simulink model "IEEE34_SPSload"  (R2021b)
settings: Solver=ode4  StartTime=0.0  StopTime=5  FixedStep=50e-6  RelTol=1e-3
PreLoadFcn:
  | pGain = 0.05; % Gain of random perturbation (pu)
  | pGainAP = 0.01; % Gain of sinusoidal active power variation (pu)
  | pGainRP = 0.01; % Gain of sinusoidal reactive power variation (pu)
  | pFreqAP = 0.03; % Frequency of sinusoidal active power variation (Hz)
  | pFreqRP = 0.03; % Frequency of sinusoidal reactive power variation (Hz)
  | 
  | init_IEEE34nodetestfeeder;
InitFcn:
  | pGain = 0.05; % Gain of random perturbation (pu)
  | pGainAP = 0.01; % Gain of sinusoidal active power variation (pu)
  | pGainRP = 0.01; % Gain of sinusoidal reactive power variation (pu)
  | pFreqAP = 0.03; % Frequency of sinusoidal active power variation (Hz)
  | pFreqRP = 0.03; % Frequency of sinusoidal reactive power variation (Hz)
  | 
  | init_IEEE34nodetestfeeder;
values from neighbouring files (symbols this model uses):
  fNom = f    (= 60)    [init_IEEE34nodetestfeeder.m]
  loadcoeff = 1.0    (= 1)    [init_IEEE34nodetestfeeder.m]
  Ts = 50e-6    (= 5e-05)    [init_IEEE34nodetestfeeder.m]
  vNomMV = VsubL    (= 24900)    [init_IEEE34nodetestfeeder.m]
  VsubL = 24.9e3    (= 24900)    [init_IEEE34nodetestfeeder.m]
  VxfmL = 4.16e3    (= 4160)    [init_IEEE34nodetestfeeder.m]
undefined symbols (not defined in the file or in its folder): Ac, Bc, Cc, Dc, find_system, j
libraries: spsSeriesRLCBranchLib x418, spsGroundLib x242, simulink_extras x176, spsVoltageMeasurementLib x106, spsRMSLib x96, spsControlledCurrentSourceLib x94, spsThreePhaseVIMeasurementLib x37, spsMutualInductanceLib x24, spsCurrentMeasurementLib x12, spsOnDelayLib x12, spsLinearTransformerLib x6, spsControlledVoltageSourceLib x6
(part 5 of 33)

== system IEEE34_SPSload/SM_IEEE34/DL836-1 ==
  Load B : Subsystem  DialogController=POWERSYS.PowerSysDialog  mask(Single-Phase Dynamic Load){NominalVoltage=[ VsubL 60 ], ActiveReactivePowers=[18*1000*loadcoeff 9*1000*loadcoeff]/2, PositiveSequence=[1 0], ExternalControl=off, NpNq=[1 1], TimeConstants=[0  0  0  0], MinimumVoltage=0.7, LoadFlowParameters=[4,0,0,0,0]}
      mask prompts: NominalVoltage "Nominal voltage and frequency  [Vn(Vrms) fn(Hz)]:"; ActiveReactivePowers "Active and reactive power at initial voltage [Po(W) Qo(var)]:"; PositiveSequence "Initial voltage Vo [Mag(pu) Phase (deg.)]:"; ExternalControl "External control of PQ"; NpNq "Parameters [ np  nq ]:"; TimeConstants "Time constants [Tp1 Tp2 Tq1 Tq2]  (s):"; MinimumVoltage "Minimum voltage Vmin (pu):"; LoadFlowParameters "Load Flow parameters"
      mask help:
      | Implements a single-phase dynamic load. Active  power P and reactive
      | power Q absorbed by the load vary as function of voltage V  according to the
      | following equations:
      |
      |   If V>Vmin, P and Q vary as follows:
      |        P = Po * (V/Vo)^np * (1+Tp1.s)/(1+Tp2.s)
      |        Q = Qo * (V/Vo)^nq * (1+Tq1.s)/(1+Tq2.s)
      |   if V<Vmin
      |      Same equations with np=nq=2 (constant impedance load)
      mask init:
      | block = gcb;
      | Ts = 50e-6;
      | %
      | Vnom=NominalVoltage(1); 
      | fnom=NominalVoltage(2);
      | P0=ActiveReactivePowers(1);
      | Q0=ActiveReactivePowers(2);
      | Mag_V0=PositiveSequence(1); 
      | Pha_V0=PositiveSequence(2);
      | V0_d=Mag_V0*cos(Pha_V0*pi/180);
      | V0_q=Mag_V0*sin(Pha_V0*pi/180);
      | np=NpNq(1);
      | nq=NpNq(2);
      | Tp1=TimeConstants(1); 
      | Tp2=TimeConstants(2); 
      | Tq1=TimeConstants(3); 
      | Tq2=TimeConstants(4);
      | Vbase=Vnom/sqrt(3)*sqrt(2);
      | % initial value of positive-sequence current I1
      | I1_init=(P0-j*Q0)/((V0_d-j*V0_q)*Vnom)/sqrt(3)*sqrt(2);
      | Mag_ia=abs(I1_init);
      | Phase_ia=angle(I1_init)*180/pi;
      | %
      | Vmin=MinimumVoltage;
      | PQext=ExternalControl;
      | a=exp(j*2*pi/3);
      | power_initmask();
      mask Help: helpview(psbhelp)
      mask Callback ExternalControl: powericon('ThreePhaseDynamicLoadCback',gcb);
      mask Display:
      | plot(-45,-45,45,45,[0,9,18,24,29,30,29,24,18,9,0,-9,-18,-24,-29,-30,-29,-24,-18,-9,0]*.9,[30,29,24,18,9,0,-9,-18,-24,-29,-30,-29,-24,-18,-9,0,9,18,24,29,30]*.9)
      | plot([0,0,10,0,-10,0]*1.1,[15,-5,-5,-15,-5,-5]*1.1)
  Load B1 : Subsystem  DialogController=POWERSYS.PowerSysDialog  mask(Single-Phase Dynamic Load){NominalVoltage=[ VsubL 60 ], ActiveReactivePowers=[22*1000*loadcoeff 11*1000*loadcoeff]/2, PositiveSequence=[1 0], ExternalControl=off, NpNq=[1 1], TimeConstants=[0  0  0  0], MinimumVoltage=0.7, LoadFlowParameters=[4,0,0,0,0]}
      mask prompts: NominalVoltage "Nominal voltage and frequency  [Vn(Vrms) fn(Hz)]:"; ActiveReactivePowers "Active and reactive power at initial voltage [Po(W) Qo(var)]:"; PositiveSequence "Initial voltage Vo [Mag(pu) Phase (deg.)]:"; ExternalControl "External control of PQ"; NpNq "Parameters [ np  nq ]:"; TimeConstants "Time constants [Tp1 Tp2 Tq1 Tq2]  (s):"; MinimumVoltage "Minimum voltage Vmin (pu):"; LoadFlowParameters "Load Flow parameters"
      mask help:
      | Implements a single-phase dynamic load. Active  power P and reactive
      | power Q absorbed by the load vary as function of voltage V  according to the
      | following equations:
      |
      |   If V>Vmin, P and Q vary as follows:
      |        P = Po * (V/Vo)^np * (1+Tp1.s)/(1+Tp2.s)
      |        Q = Qo * (V/Vo)^nq * (1+Tq1.s)/(1+Tq2.s)
      |   if V<Vmin
      |      Same equations with np=nq=2 (constant impedance load)
      mask init: same as IEEE34_SPSload/SM_IEEE34/DL836-1/Load B
      mask Help: helpview(psbhelp)
      mask Callback ExternalControl: powericon('ThreePhaseDynamicLoadCback',gcb);
      mask Display:
      | plot(-45,-45,45,45,[0,9,18,24,29,30,29,24,18,9,0,-9,-18,-24,-29,-30,-29,-24,-18,-9,0]*.9,[30,29,24,18,9,0,-9,-18,-24,-29,-30,-29,-24,-18,-9,0,9,18,24,29,30]*.9)
      | plot([0,0,10,0,-10,0]*1.1,[15,-5,-5,-15,-5,-5]*1.1)
  Load B2 : Subsystem  DialogController=POWERSYS.PowerSysDialog  mask(Single-Phase Dynamic Load){NominalVoltage=[ VsubL 60 ], ActiveReactivePowers=[1e-6*1000*loadcoeff 0*1000*loadcoeff]/2, PositiveSequence=[1 0], ExternalControl=off, NpNq=[1 1], TimeConstants=[0  0  0  0], MinimumVoltage=0.7, LoadFlowParameters=[4,0,0,0,0]}
      mask prompts: NominalVoltage "Nominal voltage and frequency  [Vn(Vrms) fn(Hz)]:"; ActiveReactivePowers "Active and reactive power at initial voltage [Po(W) Qo(var)]:"; PositiveSequence "Initial voltage Vo [Mag(pu) Phase (deg.)]:"; ExternalControl "External control of PQ"; NpNq "Parameters [ np  nq ]:"; TimeConstants "Time constants [Tp1 Tp2 Tq1 Tq2]  (s):"; MinimumVoltage "Minimum voltage Vmin (pu):"; LoadFlowParameters "Load Flow parameters"
      mask help:
      | Implements a single-phase dynamic load. Active  power P and reactive
      | power Q absorbed by the load vary as function of voltage V  according to the
      | following equations:
      |
      |   If V>Vmin, P and Q vary as follows:
      |        P = Po * (V/Vo)^np * (1+Tp1.s)/(1+Tp2.s)
      |        Q = Qo * (V/Vo)^nq * (1+Tq1.s)/(1+Tq2.s)
      |   if V<Vmin
      |      Same equations with np=nq=2 (constant impedance load)
      mask init: same as IEEE34_SPSload/SM_IEEE34/DL836-1/Load B
      mask Help: helpview(psbhelp)
      mask Callback ExternalControl: powericon('ThreePhaseDynamicLoadCback',gcb);
      mask Display:
      | plot(-45,-45,45,45,[0,9,18,24,29,30,29,24,18,9,0,-9,-18,-24,-29,-30,-29,-24,-18,-9,0]*.9,[30,29,24,18,9,0,-9,-18,-24,-29,-30,-29,-24,-18,-9,0,9,18,24,29,30]*.9)
      | plot([0,0,10,0,-10,0]*1.1,[15,-5,-5,-15,-5,-5]*1.1)
  Terminator : Terminator
  Terminator1 : Terminator
  A : PMIOPort  Side=Right
  B : PMIOPort  Port=2  Side=Right
  C : PMIOPort  Port=3  Side=Right
  wires:
  Load B1/1(m) -> Terminator1/1
  Load B/1(m) -> Terminator/1
  connections:
  C/RConn1 -- Load B1/LConn2 -- Load B2/LConn1
  Load B1/LConn1 -- Load B/LConn2 -- B/RConn1
  Load B/LConn1 -- Load B2/LConn2 -- A/RConn1

== system IEEE34_SPSload/SM_IEEE34/DL836-840 ==
  Load B : Subsystem  DialogController=POWERSYS.PowerSysDialog  mask(Single-Phase Dynamic Load){NominalVoltage=[ VsubL 60 ], ActiveReactivePowers=[18*1000*loadcoeff 9*1000*loadcoeff]/2, PositiveSequence=[1 0], ExternalControl=off, NpNq=[1 1], TimeConstants=[0  0  0  0], MinimumVoltage=0.7, LoadFlowParameters=[4,0,0,0,0]}
      mask prompts: NominalVoltage "Nominal voltage and frequency  [Vn(Vrms) fn(Hz)]:"; ActiveReactivePowers "Active and reactive power at initial voltage [Po(W) Qo(var)]:"; PositiveSequence "Initial voltage Vo [Mag(pu) Phase (deg.)]:"; ExternalControl "External control of PQ"; NpNq "Parameters [ np  nq ]:"; TimeConstants "Time constants [Tp1 Tp2 Tq1 Tq2]  (s):"; MinimumVoltage "Minimum voltage Vmin (pu):"; LoadFlowParameters "Load Flow parameters"
      mask help:
      | Implements a single-phase dynamic load. Active  power P and reactive
      | power Q absorbed by the load vary as function of voltage V  according to the
      | following equations:
      |
      |   If V>Vmin, P and Q vary as follows:
      |        P = Po * (V/Vo)^np * (1+Tp1.s)/(1+Tp2.s)
      |        Q = Qo * (V/Vo)^nq * (1+Tq1.s)/(1+Tq2.s)
      |   if V<Vmin
      |      Same equations with np=nq=2 (constant impedance load)
      mask init: same as IEEE34_SPSload/SM_IEEE34/DL836-1/Load B
      mask Help: helpview(psbhelp)
      mask Callback ExternalControl: powericon('ThreePhaseDynamicLoadCback',gcb);
      mask Display:
      | plot(-45,-45,45,45,[0,9,18,24,29,30,29,24,18,9,0,-9,-18,-24,-29,-30,-29,-24,-18,-9,0]*.9,[30,29,24,18,9,0,-9,-18,-24,-29,-30,-29,-24,-18,-9,0,9,18,24,29,30]*.9)
      | plot([0,0,10,0,-10,0]*1.1,[15,-5,-5,-15,-5,-5]*1.1)
  Load B1 : Subsystem  DialogController=POWERSYS.PowerSysDialog  mask(Single-Phase Dynamic Load){NominalVoltage=[ VsubL 60 ], ActiveReactivePowers=[22*1000*loadcoeff 11*1000*loadcoeff]/2, PositiveSequence=[1 0], ExternalControl=off, NpNq=[1 1], TimeConstants=[0  0  0  0], MinimumVoltage=0.7, LoadFlowParameters=[4,0,0,0,0]}
      mask prompts: NominalVoltage "Nominal voltage and frequency  [Vn(Vrms) fn(Hz)]:"; ActiveReactivePowers "Active and reactive power at initial voltage [Po(W) Qo(var)]:"; PositiveSequence "Initial voltage Vo [Mag(pu) Phase (deg.)]:"; ExternalControl "External control of PQ"; NpNq "Parameters [ np  nq ]:"; TimeConstants "Time constants [Tp1 Tp2 Tq1 Tq2]  (s):"; MinimumVoltage "Minimum voltage Vmin (pu):"; LoadFlowParameters "Load Flow parameters"
      mask help:
      | Implements a single-phase dynamic load. Active  power P and reactive
      | power Q absorbed by the load vary as function of voltage V  according to the
      | following equations:
      |
      |   If V>Vmin, P and Q vary as follows:
      |        P = Po * (V/Vo)^np * (1+Tp1.s)/(1+Tp2.s)
      |        Q = Qo * (V/Vo)^nq * (1+Tq1.s)/(1+Tq2.s)
      |   if V<Vmin
      |      Same equations with np=nq=2 (constant impedance load)
      mask init: same as IEEE34_SPSload/SM_IEEE34/DL836-1/Load B
      mask Help: helpview(psbhelp)
      mask Callback ExternalControl: powericon('ThreePhaseDynamicLoadCback',gcb);
      mask Display:
      | plot(-45,-45,45,45,[0,9,18,24,29,30,29,24,18,9,0,-9,-18,-24,-29,-30,-29,-24,-18,-9,0]*.9,[30,29,24,18,9,0,-9,-18,-24,-29,-30,-29,-24,-18,-9,0,9,18,24,29,30]*.9)
      | plot([0,0,10,0,-10,0]*1.1,[15,-5,-5,-15,-5,-5]*1.1)
  Load B2 : Subsystem  DialogController=POWERSYS.PowerSysDialog  mask(Single-Phase Dynamic Load){NominalVoltage=[ VsubL 60 ], ActiveReactivePowers=[1e-6*1000*loadcoeff 0*1000*loadcoeff]/2, PositiveSequence=[1 0], ExternalControl=off, NpNq=[1 1], TimeConstants=[0  0  0  0], MinimumVoltage=0.7, LoadFlowParameters=[4,0,0,0,0]}
      mask prompts: NominalVoltage "Nominal voltage and frequency  [Vn(Vrms) fn(Hz)]:"; ActiveReactivePowers "Active and reactive power at initial voltage [Po(W) Qo(var)]:"; PositiveSequence "Initial voltage Vo [Mag(pu) Phase (deg.)]:"; ExternalControl "External control of PQ"; NpNq "Parameters [ np  nq ]:"; TimeConstants "Time constants [Tp1 Tp2 Tq1 Tq2]  (s):"; MinimumVoltage "Minimum voltage Vmin (pu):"; LoadFlowParameters "Load Flow parameters"
      mask help:
      | Implements a single-phase dynamic load. Active  power P and reactive
      | power Q absorbed by the load vary as function of voltage V  according to the
      | following equations:
      |
      |   If V>Vmin, P and Q vary as follows:
      |        P = Po * (V/Vo)^np * (1+Tp1.s)/(1+Tp2.s)
      |        Q = Qo * (V/Vo)^nq * (1+Tq1.s)/(1+Tq2.s)
      |   if V<Vmin
      |      Same equations with np=nq=2 (constant impedance load)
      mask init: same as IEEE34_SPSload/SM_IEEE34/DL836-1/Load B
      mask Help: helpview(psbhelp)
      mask Callback ExternalControl: powericon('ThreePhaseDynamicLoadCback',gcb);
      mask Display:
      | plot(-45,-45,45,45,[0,9,18,24,29,30,29,24,18,9,0,-9,-18,-24,-29,-30,-29,-24,-18,-9,0]*.9,[30,29,24,18,9,0,-9,-18,-24,-29,-30,-29,-24,-18,-9,0,9,18,24,29,30]*.9)
      | plot([0,0,10,0,-10,0]*1.1,[15,-5,-5,-15,-5,-5]*1.1)
  Terminator : Terminator
  Terminator1 : Terminator
  A : PMIOPort  Side=Right
  B : PMIOPort  Port=2  Side=Right
  C : PMIOPort  Port=3  Side=Right
  wires:
  Load B/1(m) -> Terminator/1
  Load B1/1(m) -> Terminator1/1
  connections:
  A/RConn1 -- Load B2/LConn2 -- Load B/LConn1
  B/RConn1 -- Load B/LConn2 -- Load B1/LConn1
  Load B2/LConn1 -- Load B1/LConn2 -- C/RConn1

== system IEEE34_SPSload/SM_IEEE34/DL862-1 ==
  Ground3 : spsGroundLib/Ground  LConnTagsString=a
  Load B : Subsystem  DialogController=POWERSYS.PowerSysDialog  mask(Single-Phase Dynamic Load){NominalVoltage=[ VsubL/sqrt(3) 60 ], ActiveReactivePowers=[28*1000*loadcoeff 14*1000*loadcoeff]/2, PositiveSequence=[1 0], ExternalControl=off, NpNq=[0 0], TimeConstants=[0  0  0  0], MinimumVoltage=0.7, LoadFlowParameters=[4,0,0,0,0]}
      mask prompts: NominalVoltage "Nominal voltage and frequency  [Vn(Vrms) fn(Hz)]:"; ActiveReactivePowers "Active and reactive power at initial voltage [Po(W) Qo(var)]:"; PositiveSequence "Initial voltage Vo [Mag(pu) Phase (deg.)]:"; ExternalControl "External control of PQ"; NpNq "Parameters [ np  nq ]:"; TimeConstants "Time constants [Tp1 Tp2 Tq1 Tq2]  (s):"; MinimumVoltage "Minimum voltage Vmin (pu):"; LoadFlowParameters "Load Flow parameters"
      mask help:
      | Implements a single-phase dynamic load. Active  power P and reactive
      | power Q absorbed by the load vary as function of voltage V  according to the
      | following equations:
      |
      |   If V>Vmin, P and Q vary as follows:
      |        P = Po * (V/Vo)^np * (1+Tp1.s)/(1+Tp2.s)
      |        Q = Qo * (V/Vo)^nq * (1+Tq1.s)/(1+Tq2.s)
      |   if V<Vmin
      |      Same equations with np=nq=2 (constant impedance load)
      mask init: same as IEEE34_SPSload/SM_IEEE34/DL836-1/Load B
      mask Help: helpview(psbhelp)
      mask Callback ExternalControl: powericon('ThreePhaseDynamicLoadCback',gcb);
      mask Display:
      | plot(-45,-45,45,45,[0,9,18,24,29,30,29,24,18,9,0,-9,-18,-24,-29,-30,-29,-24,-18,-9,0]*.9,[30,29,24,18,9,0,-9,-18,-24,-29,-30,-29,-24,-18,-9,0,9,18,24,29,30]*.9)
      | plot([0,0,10,0,-10,0]*1.1,[15,-5,-5,-15,-5,-5]*1.1)
  Terminator : Terminator
  In : PMIOPort  Side=Right
  wires:
  Load B/1(m) -> Terminator/1
  connections:
  In/RConn1 -- Load B/LConn1
  Load B/LConn2 -- Ground3/LConn1

== system IEEE34_SPSload/SM_IEEE34/DL862-838 ==
  Ground3 : spsGroundLib/Ground  LConnTagsString=a
  Load B : Subsystem  DialogController=POWERSYS.PowerSysDialog  mask(Single-Phase Dynamic Load){NominalVoltage=[ VsubL/sqrt(3) 60 ], ActiveReactivePowers=[28*1000*loadcoeff 14*1000*loadcoeff]/2, PositiveSequence=[1 0], ExternalControl=off, NpNq=[0 0], TimeConstants=[0  0  0  0], MinimumVoltage=0.7, LoadFlowParameters=[4,0,0,0,0]}
      mask prompts: NominalVoltage "Nominal voltage and frequency  [Vn(Vrms) fn(Hz)]:"; ActiveReactivePowers "Active and reactive power at initial voltage [Po(W) Qo(var)]:"; PositiveSequence "Initial voltage Vo [Mag(pu) Phase (deg.)]:"; ExternalControl "External control of PQ"; NpNq "Parameters [ np  nq ]:"; TimeConstants "Time constants [Tp1 Tp2 Tq1 Tq2]  (s):"; MinimumVoltage "Minimum voltage Vmin (pu):"; LoadFlowParameters "Load Flow parameters"
      mask help:
      | Implements a single-phase dynamic load. Active  power P and reactive
      | power Q absorbed by the load vary as function of voltage V  according to the
      | following equations:
      |
      |   If V>Vmin, P and Q vary as follows:
      |        P = Po * (V/Vo)^np * (1+Tp1.s)/(1+Tp2.s)
      |        Q = Qo * (V/Vo)^nq * (1+Tq1.s)/(1+Tq2.s)
      |   if V<Vmin
      |      Same equations with np=nq=2 (constant impedance load)
      mask init: same as IEEE34_SPSload/SM_IEEE34/DL836-1/Load B
      mask Help: helpview(psbhelp)
      mask Callback ExternalControl: powericon('ThreePhaseDynamicLoadCback',gcb);
      mask Display:
      | plot(-45,-45,45,45,[0,9,18,24,29,30,29,24,18,9,0,-9,-18,-24,-29,-30,-29,-24,-18,-9,0]*.9,[30,29,24,18,9,0,-9,-18,-24,-29,-30,-29,-24,-18,-9,0,9,18,24,29,30]*.9)
      | plot([0,0,10,0,-10,0]*1.1,[15,-5,-5,-15,-5,-5]*1.1)
  Terminator : Terminator
  In : PMIOPort  Side=Right
  wires:
  Load B/1(m) -> Terminator/1
  connections:
  Load B/LConn2 -- Ground3/LConn1
  In/RConn1 -- Load B/LConn1

== system IEEE34_SPSload/SM_IEEE34/DL_802-1 ==
  Ground1 : spsGroundLib/Ground  LConnTagsString=a
  Ground2 : spsGroundLib/Ground  LConnTagsString=a
  Ground3 : spsGroundLib/Ground  LConnTagsString=a
  Load B : Subsystem  DialogController=POWERSYS.PowerSysDialog  mask(Single-Phase Dynamic Load){NominalVoltage=[ VsubL/sqrt(3) 60 ], ActiveReactivePowers=[30*1000*loadcoeff 15*1000*loadcoeff]/2, PositiveSequence=[1 0], ExternalControl=off, NpNq=[0 0], TimeConstants=[0  0  0  0], MinimumVoltage=0.7, LoadFlowParameters=[4,0,0,0,0]}
      mask prompts: NominalVoltage "Nominal voltage and frequency  [Vn(Vrms) fn(Hz)]:"; ActiveReactivePowers "Active and reactive power at initial voltage [Po(W) Qo(var)]:"; PositiveSequence "Initial voltage Vo [Mag(pu) Phase (deg.)]:"; ExternalControl "External control of PQ"; NpNq "Parameters [ np  nq ]:"; TimeConstants "Time constants [Tp1 Tp2 Tq1 Tq2]  (s):"; MinimumVoltage "Minimum voltage Vmin (pu):"; LoadFlowParameters "Load Flow parameters"
      mask help:
      | Implements a single-phase dynamic load. Active  power P and reactive
      | power Q absorbed by the load vary as function of voltage V  according to the
      | following equations:
      |
      |   If V>Vmin, P and Q vary as follows:
      |        P = Po * (V/Vo)^np * (1+Tp1.s)/(1+Tp2.s)
      |        Q = Qo * (V/Vo)^nq * (1+Tq1.s)/(1+Tq2.s)
      |   if V<Vmin
      |      Same equations with np=nq=2 (constant impedance load)
      mask init: same as IEEE34_SPSload/SM_IEEE34/DL836-1/Load B
      mask Help: helpview(psbhelp)
      mask Callback ExternalControl: powericon('ThreePhaseDynamicLoadCback',gcb);
      mask Display:
      | plot(-45,-45,45,45,[0,9,18,24,29,30,29,24,18,9,0,-9,-18,-24,-29,-30,-29,-24,-18,-9,0]*.9,[30,29,24,18,9,0,-9,-18,-24,-29,-30,-29,-24,-18,-9,0,9,18,24,29,30]*.9)
      | plot([0,0,10,0,-10,0]*1.1,[15,-5,-5,-15,-5,-5]*1.1)
  Load B1 : Subsystem  DialogController=POWERSYS.PowerSysDialog  mask(Single-Phase Dynamic Load){NominalVoltage=[ VsubL/sqrt(3) 60 ], ActiveReactivePowers=[1e-6*1000*loadcoeff 0*1000*loadcoeff]/2, PositiveSequence=[1 0], ExternalControl=off, NpNq=[0 0], TimeConstants=[0  0  0  0], MinimumVoltage=0.7, LoadFlowParameters=[4,0,0,0,0]}
      mask prompts: NominalVoltage "Nominal voltage and frequency  [Vn(Vrms) fn(Hz)]:"; ActiveReactivePowers "Active and reactive power at initial voltage [Po(W) Qo(var)]:"; PositiveSequence "Initial voltage Vo [Mag(pu) Phase (deg.)]:"; ExternalControl "External control of PQ"; NpNq "Parameters [ np  nq ]:"; TimeConstants "Time constants [Tp1 Tp2 Tq1 Tq2]  (s):"; MinimumVoltage "Minimum voltage Vmin (pu):"; LoadFlowParameters "Load Flow parameters"
      mask help:
      | Implements a single-phase dynamic load. Active  power P and reactive
      | power Q absorbed by the load vary as function of voltage V  according to the
      | following equations:
      |
      |   If V>Vmin, P and Q vary as follows:
      |        P = Po * (V/Vo)^np * (1+Tp1.s)/(1+Tp2.s)
      |        Q = Qo * (V/Vo)^nq * (1+Tq1.s)/(1+Tq2.s)
      |   if V<Vmin
      |      Same equations with np=nq=2 (constant impedance load)
      mask init: same as IEEE34_SPSload/SM_IEEE34/DL836-1/Load B
      mask Help: helpview(psbhelp)
      mask Callback ExternalControl: powericon('ThreePhaseDynamicLoadCback',gcb);
      mask Display:
      | plot(-45,-45,45,45,[0,9,18,24,29,30,29,24,18,9,0,-9,-18,-24,-29,-30,-29,-24,-18,-9,0]*.9,[30,29,24,18,9,0,-9,-18,-24,-29,-30,-29,-24,-18,-9,0,9,18,24,29,30]*.9)
      | plot([0,0,10,0,-10,0]*1.1,[15,-5,-5,-15,-5,-5]*1.1)
  Load C : Subsystem  DialogController=POWERSYS.PowerSysDialog  mask(Single-Phase Dynamic Load){NominalVoltage=[ VsubL/sqrt(3) 60 ], ActiveReactivePowers=[25*1000*loadcoeff 14*1000*loadcoeff]/2, PositiveSequence=[1 0], ExternalControl=off, NpNq=[0 0], TimeConstants=[0  0  0  0], MinimumVoltage=0.7, LoadFlowParameters=[4,0,0,0,0]}
      mask prompts: NominalVoltage "Nominal voltage and frequency  [Vn(Vrms) fn(Hz)]:"; ActiveReactivePowers "Active and reactive power at initial voltage [Po(W) Qo(var)]:"; PositiveSequence "Initial voltage Vo [Mag(pu) Phase (deg.)]:"; ExternalControl "External control of PQ"; NpNq "Parameters [ np  nq ]:"; TimeConstants "Time constants [Tp1 Tp2 Tq1 Tq2]  (s):"; MinimumVoltage "Minimum voltage Vmin (pu):"; LoadFlowParameters "Load Flow parameters"
      mask help:
      | Implements a single-phase dynamic load. Active  power P and reactive
      | power Q absorbed by the load vary as function of voltage V  according to the
      | following equations:
      |
      |   If V>Vmin, P and Q vary as follows:
      |        P = Po * (V/Vo)^np * (1+Tp1.s)/(1+Tp2.s)
      |        Q = Qo * (V/Vo)^nq * (1+Tq1.s)/(1+Tq2.s)
      |   if V<Vmin
      |      Same equations with np=nq=2 (constant impedance load)
      mask init: same as IEEE34_SPSload/SM_IEEE34/DL836-1/Load B
      mask Help: helpview(psbhelp)
      mask Callback ExternalControl: powericon('ThreePhaseDynamicLoadCback',gcb);
      mask Display:
      | plot(-45,-45,45,45,[0,9,18,24,29,30,29,24,18,9,0,-9,-18,-24,-29,-30,-29,-24,-18,-9,0]*.9,[30,29,24,18,9,0,-9,-18,-24,-29,-30,-29,-24,-18,-9,0,9,18,24,29,30]*.9)
      | plot([0,0,10,0,-10,0]*1.1,[15,-5,-5,-15,-5,-5]*1.1)
  Terminator : Terminator
  Terminator1 : Terminator
  Terminator2 : Terminator
  A : PMIOPort  Side=Right
  B : PMIOPort  Port=2  Side=Right
  C : PMIOPort  Port=3  Side=Right
  wires:
  Load C/1(m) -> Terminator1/1
  Load B/1(m) -> Terminator/1
  Load B1/1(m) -> Terminator2/1
  connections:
  Load C/LConn2 -- Ground1/LConn1
  Load B/LConn2 -- Ground3/LConn1
  Load C/LConn1 -- C/RConn1
  Load B/LConn1 -- B/RConn1
  Load B1/LConn1 -- A/RConn1
  Load B1/LConn2 -- Ground2/LConn1

== system IEEE34_SPSload/SM_IEEE34/DL_802-2 ==
  Ground1 : spsGroundLib/Ground  LConnTagsString=a
  Ground2 : spsGroundLib/Ground  LConnTagsString=a
  Ground3 : spsGroundLib/Ground  LConnTagsString=a
  Load B : Subsystem  DialogController=POWERSYS.PowerSysDialog  mask(Single-Phase Dynamic Load){NominalVoltage=[ VsubL/sqrt(3) 60 ], ActiveReactivePowers=[30*1000*loadcoeff 15*1000*loadcoeff]/2, PositiveSequence=[1 0], ExternalControl=off, NpNq=[0 0], TimeConstants=[0  0  0  0], MinimumVoltage=0.7, LoadFlowParameters=[4,0,0,0,0]}
      mask prompts: NominalVoltage "Nominal voltage and frequency  [Vn(Vrms) fn(Hz)]:"; ActiveReactivePowers "Active and reactive power at initial voltage [Po(W) Qo(var)]:"; PositiveSequence "Initial voltage Vo [Mag(pu) Phase (deg.)]:"; ExternalControl "External control of PQ"; NpNq "Parameters [ np  nq ]:"; TimeConstants "Time constants [Tp1 Tp2 Tq1 Tq2]  (s):"; MinimumVoltage "Minimum voltage Vmin (pu):"; LoadFlowParameters "Load Flow parameters"
      mask help:
      | Implements a single-phase dynamic load. Active  power P and reactive
      | power Q absorbed by the load vary as function of voltage V  according to the
      | following equations:
      |
      |   If V>Vmin, P and Q vary as follows:
      |        P = Po * (V/Vo)^np * (1+Tp1.s)/(1+Tp2.s)
      |        Q = Qo * (V/Vo)^nq * (1+Tq1.s)/(1+Tq2.s)
      |   if V<Vmin
      |      Same equations with np=nq=2 (constant impedance load)
      mask init: same as IEEE34_SPSload/SM_IEEE34/DL836-1/Load B
      mask Help: helpview(psbhelp)
      mask Callback ExternalControl: powericon('ThreePhaseDynamicLoadCback',gcb);
      mask Display:
      | plot(-45,-45,45,45,[0,9,18,24,29,30,29,24,18,9,0,-9,-18,-24,-29,-30,-29,-24,-18,-9,0]*.9,[30,29,24,18,9,0,-9,-18,-24,-29,-30,-29,-24,-18,-9,0,9,18,24,29,30]*.9)
      | plot([0,0,10,0,-10,0]*1.1,[15,-5,-5,-15,-5,-5]*1.1)
  Load B1 : Subsystem  DialogController=POWERSYS.PowerSysDialog  mask(Single-Phase Dynamic Load){NominalVoltage=[ VsubL/sqrt(3) 60 ], ActiveReactivePowers=[1e-6*1000*loadcoeff 0*1000*loadcoeff]/2, PositiveSequence=[1 0], ExternalControl=off, NpNq=[0 0], TimeConstants=[0  0  0  0], MinimumVoltage=0.7, LoadFlowParameters=[4,0,0,0,0]}
      mask prompts: NominalVoltage "Nominal voltage and frequency  [Vn(Vrms) fn(Hz)]:"; ActiveReactivePowers "Active and reactive power at initial voltage [Po(W) Qo(var)]:"; PositiveSequence "Initial voltage Vo [Mag(pu) Phase (deg.)]:"; ExternalControl "External control of PQ"; NpNq "Parameters [ np  nq ]:"; TimeConstants "Time constants [Tp1 Tp2 Tq1 Tq2]  (s):"; MinimumVoltage "Minimum voltage Vmin (pu):"; LoadFlowParameters "Load Flow parameters"
      mask help:
      | Implements a single-phase dynamic load. Active  power P and reactive
      | power Q absorbed by the load vary as function of voltage V  according to the
      | following equations:
      |
      |   If V>Vmin, P and Q vary as follows:
      |        P = Po * (V/Vo)^np * (1+Tp1.s)/(1+Tp2.s)
      |        Q = Qo * (V/Vo)^nq * (1+Tq1.s)/(1+Tq2.s)
      |   if V<Vmin
      |      Same equations with np=nq=2 (constant impedance load)
      mask init: same as IEEE34_SPSload/SM_IEEE34/DL836-1/Load B
      mask Help: helpview(psbhelp)
      mask Callback ExternalControl: powericon('ThreePhaseDynamicLoadCback',gcb);
      mask Display:
      | plot(-45,-45,45,45,[0,9,18,24,29,30,29,24,18,9,0,-9,-18,-24,-29,-30,-29,-24,-18,-9,0]*.9,[30,29,24,18,9,0,-9,-18,-24,-29,-30,-29,-24,-18,-9,0,9,18,24,29,30]*.9)
      | plot([0,0,10,0,-10,0]*1.1,[15,-5,-5,-15,-5,-5]*1.1)
  Load C : Subsystem  DialogController=POWERSYS.PowerSysDialog  mask(Single-Phase Dynamic Load){NominalVoltage=[ VsubL/sqrt(3) 60 ], ActiveReactivePowers=[25*1000*loadcoeff 14*1000*loadcoeff]/2, PositiveSequence=[1 0], ExternalControl=off, NpNq=[0 0], TimeConstants=[0  0  0  0], MinimumVoltage=0.7, LoadFlowParameters=[4,0,0,0,0]}
      mask prompts: NominalVoltage "Nominal voltage and frequency  [Vn(Vrms) fn(Hz)]:"; ActiveReactivePowers "Active and reactive power at initial voltage [Po(W) Qo(var)]:"; PositiveSequence "Initial voltage Vo [Mag(pu) Phase (deg.)]:"; ExternalControl "External control of PQ"; NpNq "Parameters [ np  nq ]:"; TimeConstants "Time constants [Tp1 Tp2 Tq1 Tq2]  (s):"; MinimumVoltage "Minimum voltage Vmin (pu):"; LoadFlowParameters "Load Flow parameters"
      mask help:
      | Implements a single-phase dynamic load. Active  power P and reactive
      | power Q absorbed by the load vary as function of voltage V  according to the
      | following equations:
      |
      |   If V>Vmin, P and Q vary as follows:
      |        P = Po * (V/Vo)^np * (1+Tp1.s)/(1+Tp2.s)
      |        Q = Qo * (V/Vo)^nq * (1+Tq1.s)/(1+Tq2.s)
      |   if V<Vmin
      |      Same equations with np=nq=2 (constant impedance load)
      mask init: same as IEEE34_SPSload/SM_IEEE34/DL836-1/Load B
      mask Help: helpview(psbhelp)
      mask Callback ExternalControl: powericon('ThreePhaseDynamicLoadCback',gcb);
      mask Display:
      | plot(-45,-45,45,45,[0,9,18,24,29,30,29,24,18,9,0,-9,-18,-24,-29,-30,-29,-24,-18,-9,0]*.9,[30,29,24,18,9,0,-9,-18,-24,-29,-30,-29,-24,-18,-9,0,9,18,24,29,30]*.9)
      | plot([0,0,10,0,-10,0]*1.1,[15,-5,-5,-15,-5,-5]*1.1)
  Terminator : Terminator
  Terminator1 : Terminator
  Terminator2 : Terminator
  A : PMIOPort  Side=Right
  B : PMIOPort  Port=2  Side=Right
  C : PMIOPort  Port=3  Side=Right
  wires:
  Load B1/1(m) -> Terminator2/1
  Load B/1(m) -> Terminator/1
  Load C/1(m) -> Terminator1/1
  connections:
  Load B1/LConn2 -- Ground2/LConn1
  Load B1/LConn1 -- A/RConn1
  Load B/LConn1 -- B/RConn1
  Load C/LConn1 -- C/RConn1
  Load B/LConn2 -- Ground3/LConn1
  Load C/LConn2 -- Ground1/LConn1

== system IEEE34_SPSload/SM_IEEE34/DL_808-1 ==
  Ground3 : spsGroundLib/Ground  LConnTagsString=a
  Load B : Subsystem  DialogController=POWERSYS.PowerSysDialog  mask(Single-Phase Dynamic Load){NominalVoltage=[ VsubL/sqrt(3) 60 ], ActiveReactivePowers=[16*1000*loadcoeff 8*1000*loadcoeff]/2, PositiveSequence=[1 0], ExternalControl=off, NpNq=[1 1], TimeConstants=[0  0  0  0], MinimumVoltage=0.7, LoadFlowParameters=[4,0,0,0,0]}
      mask prompts: NominalVoltage "Nominal voltage and frequency  [Vn(Vrms) fn(Hz)]:"; ActiveReactivePowers "Active and reactive power at initial voltage [Po(W) Qo(var)]:"; PositiveSequence "Initial voltage Vo [Mag(pu) Phase (deg.)]:"; ExternalControl "External control of PQ"; NpNq "Parameters [ np  nq ]:"; TimeConstants "Time constants [Tp1 Tp2 Tq1 Tq2]  (s):"; MinimumVoltage "Minimum voltage Vmin (pu):"; LoadFlowParameters "Load Flow parameters"
      mask help:
      | Implements a single-phase dynamic load. Active  power P and reactive
      | power Q absorbed by the load vary as function of voltage V  according to the
      | following equations:
      |
      |   If V>Vmin, P and Q vary as follows:
      |        P = Po * (V/Vo)^np * (1+Tp1.s)/(1+Tp2.s)
      |        Q = Qo * (V/Vo)^nq * (1+Tq1.s)/(1+Tq2.s)
      |   if V<Vmin
      |      Same equations with np=nq=2 (constant impedance load)
      mask init: same as IEEE34_SPSload/SM_IEEE34/DL836-1/Load B
      mask Help: helpview(psbhelp)
      mask Callback ExternalControl: powericon('ThreePhaseDynamicLoadCback',gcb);
      mask Display:
      | plot(-45,-45,45,45,[0,9,18,24,29,30,29,24,18,9,0,-9,-18,-24,-29,-30,-29,-24,-18,-9,0]*.9,[30,29,24,18,9,0,-9,-18,-24,-29,-30,-29,-24,-18,-9,0,9,18,24,29,30]*.9)
      | plot([0,0,10,0,-10,0]*1.1,[15,-5,-5,-15,-5,-5]*1.1)
  Terminator : Terminator
  In : PMIOPort  Side=Right
  wires:
  Load B/1(m) -> Terminator/1
  connections:
  Load B/LConn2 -- Ground3/LConn1
  In/RConn1 -- Load B/LConn1

== system IEEE34_SPSload/SM_IEEE34/DL_808-810 ==
  Ground3 : spsGroundLib/Ground  LConnTagsString=a
  Load B : Subsystem  DialogController=POWERSYS.PowerSysDialog  mask(Single-Phase Dynamic Load){NominalVoltage=[ VsubL/sqrt(3) 60 ], ActiveReactivePowers=[16*1000*loadcoeff 8*1000*loadcoeff]/2, PositiveSequence=[1 0], ExternalControl=off, NpNq=[1 1], TimeConstants=[0  0  0  0], MinimumVoltage=0.7, LoadFlowParameters=[4,0,0,0,0]}
      mask prompts: NominalVoltage "Nominal voltage and frequency  [Vn(Vrms) fn(Hz)]:"; ActiveReactivePowers "Active and reactive power at initial voltage [Po(W) Qo(var)]:"; PositiveSequence "Initial voltage Vo [Mag(pu) Phase (deg.)]:"; ExternalControl "External control of PQ"; NpNq "Parameters [ np  nq ]:"; TimeConstants "Time constants [Tp1 Tp2 Tq1 Tq2]  (s):"; MinimumVoltage "Minimum voltage Vmin (pu):"; LoadFlowParameters "Load Flow parameters"
      mask help:
      | Implements a single-phase dynamic load. Active  power P and reactive
      | power Q absorbed by the load vary as function of voltage V  according to the
      | following equations:
      |
      |   If V>Vmin, P and Q vary as follows:
      |        P = Po * (V/Vo)^np * (1+Tp1.s)/(1+Tp2.s)
      |        Q = Qo * (V/Vo)^nq * (1+Tq1.s)/(1+Tq2.s)
      |   if V<Vmin
      |      Same equations with np=nq=2 (constant impedance load)
      mask init: same as IEEE34_SPSload/SM_IEEE34/DL836-1/Load B
      mask Help: helpview(psbhelp)
      mask Callback ExternalControl: powericon('ThreePhaseDynamicLoadCback',gcb);
      mask Display:
      | plot(-45,-45,45,45,[0,9,18,24,29,30,29,24,18,9,0,-9,-18,-24,-29,-30,-29,-24,-18,-9,0]*.9,[30,29,24,18,9,0,-9,-18,-24,-29,-30,-29,-24,-18,-9,0,9,18,24,29,30]*.9)
      | plot([0,0,10,0,-10,0]*1.1,[15,-5,-5,-15,-5,-5]*1.1)
  Terminator : Terminator
  In : PMIOPort  Side=Right
  wires:
  Load B/1(m) -> Terminator/1
  connections:
  In/RConn1 -- Load B/LConn1
  Load B/LConn2 -- Ground3/LConn1

== system IEEE34_SPSload/SM_IEEE34/DL_816-1 ==
  Load B : Subsystem  DialogController=POWERSYS.PowerSysDialog  mask(Single-Phase Dynamic Load){NominalVoltage=[ VsubL 60 ], ActiveReactivePowers=[5*1000*loadcoeff 2*1000*loadcoeff]/2, PositiveSequence=[1 0], ExternalControl=off, NpNq=[1 1], TimeConstants=[0  0  0  0], MinimumVoltage=0.7, LoadFlowParameters=[4,0,0,0,0]}
      mask prompts: NominalVoltage "Nominal voltage and frequency  [Vn(Vrms) fn(Hz)]:"; ActiveReactivePowers "Active and reactive power at initial voltage [Po(W) Qo(var)]:"; PositiveSequence "Initial voltage Vo [Mag(pu) Phase (deg.)]:"; ExternalControl "External control of PQ"; NpNq "Parameters [ np  nq ]:"; TimeConstants "Time constants [Tp1 Tp2 Tq1 Tq2]  (s):"; MinimumVoltage "Minimum voltage Vmin (pu):"; LoadFlowParameters "Load Flow parameters"
      mask help:
      | Implements a single-phase dynamic load. Active  power P and reactive
      | power Q absorbed by the load vary as function of voltage V  according to the
      | following equations:
      |
      |   If V>Vmin, P and Q vary as follows:
      |        P = Po * (V/Vo)^np * (1+Tp1.s)/(1+Tp2.s)
      |        Q = Qo * (V/Vo)^nq * (1+Tq1.s)/(1+Tq2.s)
      |   if V<Vmin
      |      Same equations with np=nq=2 (constant impedance load)
      mask init: same as IEEE34_SPSload/SM_IEEE34/DL836-1/Load B
      mask Help: helpview(psbhelp)
      mask Callback ExternalControl: powericon('ThreePhaseDynamicLoadCback',gcb);
      mask Display:
      | plot(-45,-45,45,45,[0,9,18,24,29,30,29,24,18,9,0,-9,-18,-24,-29,-30,-29,-24,-18,-9,0]*.9,[30,29,24,18,9,0,-9,-18,-24,-29,-30,-29,-24,-18,-9,0,9,18,24,29,30]*.9)
      | plot([0,0,10,0,-10,0]*1.1,[15,-5,-5,-15,-5,-5]*1.1)
  Load B1 : Subsystem  DialogController=POWERSYS.PowerSysDialog  mask(Single-Phase Dynamic Load){NominalVoltage=[ VsubL 60 ], ActiveReactivePowers=[1e-6*1000*loadcoeff 0*1000*loadcoeff]/2, PositiveSequence=[1 0], ExternalControl=off, NpNq=[1 1], TimeConstants=[0  0  0  0], MinimumVoltage=0.7, LoadFlowParameters=[4,0,0,0,0]}
      mask prompts: NominalVoltage "Nominal voltage and frequency  [Vn(Vrms) fn(Hz)]:"; ActiveReactivePowers "Active and reactive power at initial voltage [Po(W) Qo(var)]:"; PositiveSequence "Initial voltage Vo [Mag(pu) Phase (deg.)]:"; ExternalControl "External control of PQ"; NpNq "Parameters [ np  nq ]:"; TimeConstants "Time constants [Tp1 Tp2 Tq1 Tq2]  (s):"; MinimumVoltage "Minimum voltage Vmin (pu):"; LoadFlowParameters "Load Flow parameters"
      mask help:
      | Implements a single-phase dynamic load. Active  power P and reactive
      | power Q absorbed by the load vary as function of voltage V  according to the
      | following equations:
      |
      |   If V>Vmin, P and Q vary as follows:
      |        P = Po * (V/Vo)^np * (1+Tp1.s)/(1+Tp2.s)
      |        Q = Qo * (V/Vo)^nq * (1+Tq1.s)/(1+Tq2.s)
      |   if V<Vmin
      |      Same equations with np=nq=2 (constant impedance load)
      mask init: same as IEEE34_SPSload/SM_IEEE34/DL836-1/Load B
      mask Help: helpview(psbhelp)
      mask Callback ExternalControl: powericon('ThreePhaseDynamicLoadCback',gcb);
      mask Display:
      | plot(-45,-45,45,45,[0,9,18,24,29,30,29,24,18,9,0,-9,-18,-24,-29,-30,-29,-24,-18,-9,0]*.9,[30,29,24,18,9,0,-9,-18,-24,-29,-30,-29,-24,-18,-9,0,9,18,24,29,30]*.9)
      | plot([0,0,10,0,-10,0]*1.1,[15,-5,-5,-15,-5,-5]*1.1)
  Load B2 : Subsystem  DialogController=POWERSYS.PowerSysDialog  mask(Single-Phase Dynamic Load){NominalVoltage=[ VsubL 60 ], ActiveReactivePowers=[1e-6*1000*loadcoeff 0*1000*loadcoeff]/2, PositiveSequence=[1 0], ExternalControl=off, NpNq=[1 1], TimeConstants=[0  0  0  0], MinimumVoltage=0.7, LoadFlowParameters=[4,0,0,0,0]}
      mask prompts: NominalVoltage "Nominal voltage and frequency  [Vn(Vrms) fn(Hz)]:"; ActiveReactivePowers "Active and reactive power at initial voltage [Po(W) Qo(var)]:"; PositiveSequence "Initial voltage Vo [Mag(pu) Phase (deg.)]:"; ExternalControl "External control of PQ"; NpNq "Parameters [ np  nq ]:"; TimeConstants "Time constants [Tp1 Tp2 Tq1 Tq2]  (s):"; MinimumVoltage "Minimum voltage Vmin (pu):"; LoadFlowParameters "Load Flow parameters"
      mask help:
      | Implements a single-phase dynamic load. Active  power P and reactive
      | power Q absorbed by the load vary as function of voltage V  according to the
      | following equations:
      |
      |   If V>Vmin, P and Q vary as follows:
      |        P = Po * (V/Vo)^np * (1+Tp1.s)/(1+Tp2.s)
      |        Q = Qo * (V/Vo)^nq * (1+Tq1.s)/(1+Tq2.s)
      |   if V<Vmin
      |      Same equations with np=nq=2 (constant impedance load)
      mask init: same as IEEE34_SPSload/SM_IEEE34/DL836-1/Load B
      mask Help: helpview(psbhelp)
      mask Callback ExternalControl: powericon('ThreePhaseDynamicLoadCback',gcb);
      mask Display:
      | plot(-45,-45,45,45,[0,9,18,24,29,30,29,24,18,9,0,-9,-18,-24,-29,-30,-29,-24,-18,-9,0]*.9,[30,29,24,18,9,0,-9,-18,-24,-29,-30,-29,-24,-18,-9,0,9,18,24,29,30]*.9)
      | plot([0,0,10,0,-10,0]*1.1,[15,-5,-5,-15,-5,-5]*1.1)
  Terminator : Terminator
  Terminator1 : Terminator
  Terminator2 : Terminator
  A : PMIOPort  Side=Right
  B : PMIOPort  Port=2  Side=Right
  C : PMIOPort  Port=3  Side=Right
  wires:
  Load B/1(m) -> Terminator/1
  Load B1/1(m) -> Terminator1/1
  Load B2/1(m) -> Terminator2/1
  connections:
  A/RConn1 -- Load B2/LConn2 -- Load B1/LConn1
  B/RConn1 -- Load B1/LConn2 -- Load B/LConn1
  C/RConn1 -- Load B/LConn2 -- Load B2/LConn1

== system IEEE34_SPSload/SM_IEEE34/DL_816-824 ==
  Load B : Subsystem  DialogController=POWERSYS.PowerSysDialog  mask(Single-Phase Dynamic Load){NominalVoltage=[ VsubL 60 ], ActiveReactivePowers=[5*1000*loadcoeff 2*1000*loadcoeff]/2, PositiveSequence=[1 0], ExternalControl=off, NpNq=[1 1], TimeConstants=[0  0  0  0], MinimumVoltage=0.7, LoadFlowParameters=[4,0,0,0,0]}
      mask prompts: NominalVoltage "Nominal voltage and frequency  [Vn(Vrms) fn(Hz)]:"; ActiveReactivePowers "Active and reactive power at initial voltage [Po(W) Qo(var)]:"; PositiveSequence "Initial voltage Vo [Mag(pu) Phase (deg.)]:"; ExternalControl "External control of PQ"; NpNq "Parameters [ np  nq ]:"; TimeConstants "Time constants [Tp1 Tp2 Tq1 Tq2]  (s):"; MinimumVoltage "Minimum voltage Vmin (pu):"; LoadFlowParameters "Load Flow parameters"
      mask help:
      | Implements a single-phase dynamic load. Active  power P and reactive
      | power Q absorbed by the load vary as function of voltage V  according to the
      | following equations:
      |
      |   If V>Vmin, P and Q vary as follows:
      |        P = Po * (V/Vo)^np * (1+Tp1.s)/(1+Tp2.s)
      |        Q = Qo * (V/Vo)^nq * (1+Tq1.s)/(1+Tq2.s)
      |   if V<Vmin
      |      Same equations with np=nq=2 (constant impedance load)
      mask init: same as IEEE34_SPSload/SM_IEEE34/DL836-1/Load B
      mask Help: helpview(psbhelp)
      mask Callback ExternalControl: powericon('ThreePhaseDynamicLoadCback',gcb);
      mask Display:
      | plot(-45,-45,45,45,[0,9,18,24,29,30,29,24,18,9,0,-9,-18,-24,-29,-30,-29,-24,-18,-9,0]*.9,[30,29,24,18,9,0,-9,-18,-24,-29,-30,-29,-24,-18,-9,0,9,18,24,29,30]*.9)
      | plot([0,0,10,0,-10,0]*1.1,[15,-5,-5,-15,-5,-5]*1.1)
  Load B1 : Subsystem  DialogController=POWERSYS.PowerSysDialog  mask(Single-Phase Dynamic Load){NominalVoltage=[ VsubL 60 ], ActiveReactivePowers=[1e-6*1000*loadcoeff 0*1000*loadcoeff]/2, PositiveSequence=[1 0], ExternalControl=off, NpNq=[1 1], TimeConstants=[0  0  0  0], MinimumVoltage=0.7, LoadFlowParameters=[4,0,0,0,0]}
      mask prompts: NominalVoltage "Nominal voltage and frequency  [Vn(Vrms) fn(Hz)]:"; ActiveReactivePowers "Active and reactive power at initial voltage [Po(W) Qo(var)]:"; PositiveSequence "Initial voltage Vo [Mag(pu) Phase (deg.)]:"; ExternalControl "External control of PQ"; NpNq "Parameters [ np  nq ]:"; TimeConstants "Time constants [Tp1 Tp2 Tq1 Tq2]  (s):"; MinimumVoltage "Minimum voltage Vmin (pu):"; LoadFlowParameters "Load Flow parameters"
      mask help:
      | Implements a single-phase dynamic load. Active  power P and reactive
      | power Q absorbed by the load vary as function of voltage V  according to the
      | following equations:
      |
      |   If V>Vmin, P and Q vary as follows:
      |        P = Po * (V/Vo)^np * (1+Tp1.s)/(1+Tp2.s)
      |        Q = Qo * (V/Vo)^nq * (1+Tq1.s)/(1+Tq2.s)
      |   if V<Vmin
      |      Same equations with np=nq=2 (constant impedance load)
      mask init: same as IEEE34_SPSload/SM_IEEE34/DL836-1/Load B
      mask Help: helpview(psbhelp)
      mask Callback ExternalControl: powericon('ThreePhaseDynamicLoadCback',gcb);
      mask Display:
      | plot(-45,-45,45,45,[0,9,18,24,29,30,29,24,18,9,0,-9,-18,-24,-29,-30,-29,-24,-18,-9,0]*.9,[30,29,24,18,9,0,-9,-18,-24,-29,-30,-29,-24,-18,-9,0,9,18,24,29,30]*.9)
      | plot([0,0,10,0,-10,0]*1.1,[15,-5,-5,-15,-5,-5]*1.1)
  Load B2 : Subsystem  DialogController=POWERSYS.PowerSysDialog  mask(Single-Phase Dynamic Load){NominalVoltage=[ VsubL 60 ], ActiveReactivePowers=[1e-6*1000*loadcoeff 0*1000*loadcoeff]/2, PositiveSequence=[1 0], ExternalControl=off, NpNq=[1 1], TimeConstants=[0  0  0  0], MinimumVoltage=0.7, LoadFlowParameters=[4,0,0,0,0]}
      mask prompts: NominalVoltage "Nominal voltage and frequency  [Vn(Vrms) fn(Hz)]:"; ActiveReactivePowers "Active and reactive power at initial voltage [Po(W) Qo(var)]:"; PositiveSequence "Initial voltage Vo [Mag(pu) Phase (deg.)]:"; ExternalControl "External control of PQ"; NpNq "Parameters [ np  nq ]:"; TimeConstants "Time constants [Tp1 Tp2 Tq1 Tq2]  (s):"; MinimumVoltage "Minimum voltage Vmin (pu):"; LoadFlowParameters "Load Flow parameters"
      mask help:
      | Implements a single-phase dynamic load. Active  power P and reactive
      | power Q absorbed by the load vary as function of voltage V  according to the
      | following equations:
      |
      |   If V>Vmin, P and Q vary as follows:
      |        P = Po * (V/Vo)^np * (1+Tp1.s)/(1+Tp2.s)
      |        Q = Qo * (V/Vo)^nq * (1+Tq1.s)/(1+Tq2.s)
      |   if V<Vmin
      |      Same equations with np=nq=2 (constant impedance load)
      mask init: same as IEEE34_SPSload/SM_IEEE34/DL836-1/Load B
      mask Help: helpview(psbhelp)
      mask Callback ExternalControl: powericon('ThreePhaseDynamicLoadCback',gcb);
      mask Display:
      | plot(-45,-45,45,45,[0,9,18,24,29,30,29,24,18,9,0,-9,-18,-24,-29,-30,-29,-24,-18,-9,0]*.9,[30,29,24,18,9,0,-9,-18,-24,-29,-30,-29,-24,-18,-9,0,9,18,24,29,30]*.9)
      | plot([0,0,10,0,-10,0]*1.1,[15,-5,-5,-15,-5,-5]*1.1)
  Terminator : Terminator
  Terminator1 : Terminator
  Terminator2 : Terminator
  A : PMIOPort  Side=Right
  B : PMIOPort  Port=2  Side=Right
  C : PMIOPort  Port=3  Side=Right
  wires:
  Load B2/1(m) -> Terminator2/1
  Load B1/1(m) -> Terminator1/1
  Load B/1(m) -> Terminator/1
  connections:
  Load B/LConn2 -- C/RConn1 -- Load B2/LConn1
  Load B1/LConn2 -- B/RConn1 -- Load B/LConn1
  Load B2/LConn2 -- A/RConn1 -- Load B1/LConn1

== system IEEE34_SPSload/SM_IEEE34/DL_818-1 ==
  Ground3 : spsGroundLib/Ground  LConnTagsString=a
  Load B : Subsystem  DialogController=POWERSYS.PowerSysDialog  mask(Single-Phase Dynamic Load){NominalVoltage=[ VsubL/sqrt(3) 60 ], ActiveReactivePowers=[34*1000*loadcoeff 17*1000*loadcoeff]/2, PositiveSequence=[1 0], ExternalControl=off, NpNq=[2 2], TimeConstants=[0  0  0  0], MinimumVoltage=0.7, LoadFlowParameters=[4,0,0,0,0]}
      mask prompts: NominalVoltage "Nominal voltage and frequency  [Vn(Vrms) fn(Hz)]:"; ActiveReactivePowers "Active and reactive power at initial voltage [Po(W) Qo(var)]:"; PositiveSequence "Initial voltage Vo [Mag(pu) Phase (deg.)]:"; ExternalControl "External control of PQ"; NpNq "Parameters [ np  nq ]:"; TimeConstants "Time constants [Tp1 Tp2 Tq1 Tq2]  (s):"; MinimumVoltage "Minimum voltage Vmin (pu):"; LoadFlowParameters "Load Flow parameters"
      mask help:
      | Implements a single-phase dynamic load. Active  power P and reactive
      | power Q absorbed by the load vary as function of voltage V  according to the
      | following equations:
      |
      |   If V>Vmin, P and Q vary as follows:
      |        P = Po * (V/Vo)^np * (1+Tp1.s)/(1+Tp2.s)
      |        Q = Qo * (V/Vo)^nq * (1+Tq1.s)/(1+Tq2.s)
      |   if V<Vmin
      |      Same equations with np=nq=2 (constant impedance load)
      mask init: same as IEEE34_SPSload/SM_IEEE34/DL836-1/Load B
      mask Help: helpview(psbhelp)
      mask Callback ExternalControl: powericon('ThreePhaseDynamicLoadCback',gcb);
      mask Display:
      | plot(-45,-45,45,45,[0,9,18,24,29,30,29,24,18,9,0,-9,-18,-24,-29,-30,-29,-24,-18,-9,0]*.9,[30,29,24,18,9,0,-9,-18,-24,-29,-30,-29,-24,-18,-9,0,9,18,24,29,30]*.9)
      | plot([0,0,10,0,-10,0]*1.1,[15,-5,-5,-15,-5,-5]*1.1)
  Terminator : Terminator
  In : PMIOPort  Side=Right
  wires:
  Load B/1(m) -> Terminator/1
  connections:
  Load B/LConn2 -- Ground3/LConn1
  In/RConn1 -- Load B/LConn1

== system IEEE34_SPSload/SM_IEEE34/DL_818-820 ==
  Ground3 : spsGroundLib/Ground  LConnTagsString=a
  Load B : Subsystem  DialogController=POWERSYS.PowerSysDialog  mask(Single-Phase Dynamic Load){NominalVoltage=[ VsubL/sqrt(3) 60 ], ActiveReactivePowers=[34*1000*loadcoeff 17*1000*loadcoeff]/2, PositiveSequence=[1 0], ExternalControl=off, NpNq=[2 2], TimeConstants=[0  0  0  0], MinimumVoltage=0.7, LoadFlowParameters=[4,0,0,0,0]}
      mask prompts: NominalVoltage "Nominal voltage and frequency  [Vn(Vrms) fn(Hz)]:"; ActiveReactivePowers "Active and reactive power at initial voltage [Po(W) Qo(var)]:"; PositiveSequence "Initial voltage Vo [Mag(pu) Phase (deg.)]:"; ExternalControl "External control of PQ"; NpNq "Parameters [ np  nq ]:"; TimeConstants "Time constants [Tp1 Tp2 Tq1 Tq2]  (s):"; MinimumVoltage "Minimum voltage Vmin (pu):"; LoadFlowParameters "Load Flow parameters"
      mask help:
      | Implements a single-phase dynamic load. Active  power P and reactive
      | power Q absorbed by the load vary as function of voltage V  according to the
      | following equations:
      |
      |   If V>Vmin, P and Q vary as follows:
      |        P = Po * (V/Vo)^np * (1+Tp1.s)/(1+Tp2.s)
      |        Q = Qo * (V/Vo)^nq * (1+Tq1.s)/(1+Tq2.s)
      |   if V<Vmin
      |      Same equations with np=nq=2 (constant impedance load)
      mask init: same as IEEE34_SPSload/SM_IEEE34/DL836-1/Load B
      mask Help: helpview(psbhelp)
      mask Callback ExternalControl: powericon('ThreePhaseDynamicLoadCback',gcb);
      mask Display:
      | plot(-45,-45,45,45,[0,9,18,24,29,30,29,24,18,9,0,-9,-18,-24,-29,-30,-29,-24,-18,-9,0]*.9,[30,29,24,18,9,0,-9,-18,-24,-29,-30,-29,-24,-18,-9,0,9,18,24,29,30]*.9)
      | plot([0,0,10,0,-10,0]*1.1,[15,-5,-5,-15,-5,-5]*1.1)
  Terminator : Terminator
  In : PMIOPort  Side=Right
  wires:
  Load B/1(m) -> Terminator/1
  connections:
  In/RConn1 -- Load B/LConn1
  Load B/LConn2 -- Ground3/LConn1

== system IEEE34_SPSload/SM_IEEE34/DL_820-1 ==
  Ground3 : spsGroundLib/Ground  LConnTagsString=a
  Load B : Subsystem  DialogController=POWERSYS.PowerSysDialog  mask(Single-Phase Dynamic Load){NominalVoltage=[ VsubL/sqrt(3) 60 ], ActiveReactivePowers=[135*1000*loadcoeff 70*1000*loadcoeff]/2, PositiveSequence=[1 0], ExternalControl=off, NpNq=[0 0], TimeConstants=[0  0  0  0], MinimumVoltage=0.7, LoadFlowParameters=[4,0,0,0,0]}
      mask prompts: NominalVoltage "Nominal voltage and frequency  [Vn(Vrms) fn(Hz)]:"; ActiveReactivePowers "Active and reactive power at initial voltage [Po(W) Qo(var)]:"; PositiveSequence "Initial voltage Vo [Mag(pu) Phase (deg.)]:"; ExternalControl "External control of PQ"; NpNq "Parameters [ np  nq ]:"; TimeConstants "Time constants [Tp1 Tp2 Tq1 Tq2]  (s):"; MinimumVoltage "Minimum voltage Vmin (pu):"; LoadFlowParameters "Load Flow parameters"
      mask help:
      | Implements a single-phase dynamic load. Active  power P and reactive
      | power Q absorbed by the load vary as function of voltage V  according to the
      | following equations:
      |
      |   If V>Vmin, P and Q vary as follows:
      |        P = Po * (V/Vo)^np * (1+Tp1.s)/(1+Tp2.s)
      |        Q = Qo * (V/Vo)^nq * (1+Tq1.s)/(1+Tq2.s)
      |   if V<Vmin
      |      Same equations with np=nq=2 (constant impedance load)
      mask init: same as IEEE34_SPSload/SM_IEEE34/DL836-1/Load B
      mask Help: helpview(psbhelp)
      mask Callback ExternalControl: powericon('ThreePhaseDynamicLoadCback',gcb);
      mask Display:
      | plot(-45,-45,45,45,[0,9,18,24,29,30,29,24,18,9,0,-9,-18,-24,-29,-30,-29,-24,-18,-9,0]*.9,[30,29,24,18,9,0,-9,-18,-24,-29,-30,-29,-24,-18,-9,0,9,18,24,29,30]*.9)
      | plot([0,0,10,0,-10,0]*1.1,[15,-5,-5,-15,-5,-5]*1.1)
  Terminator : Terminator
  In : PMIOPort  Side=Right
  wires:
  Load B/1(m) -> Terminator/1
  connections:
  Load B/LConn2 -- Ground3/LConn1
  In/RConn1 -- Load B/LConn1

== system IEEE34_SPSload/SM_IEEE34/DL_820-822 ==
  Ground3 : spsGroundLib/Ground  LConnTagsString=a
  Load B : Subsystem  DialogController=POWERSYS.PowerSysDialog  mask(Single-Phase Dynamic Load){NominalVoltage=[ VsubL/sqrt(3) 60 ], ActiveReactivePowers=[135*1000*loadcoeff 70*1000*loadcoeff]/2, PositiveSequence=[1 0], ExternalControl=off, NpNq=[0 0], TimeConstants=[0  0  0  0], MinimumVoltage=0.7, LoadFlowParameters=[4,0,0,0,0]}
      mask prompts: NominalVoltage "Nominal voltage and frequency  [Vn(Vrms) fn(Hz)]:"; ActiveReactivePowers "Active and reactive power at initial voltage [Po(W) Qo(var)]:"; PositiveSequence "Initial voltage Vo [Mag(pu) Phase (deg.)]:"; ExternalControl "External control of PQ"; NpNq "Parameters [ np  nq ]:"; TimeConstants "Time constants [Tp1 Tp2 Tq1 Tq2]  (s):"; MinimumVoltage "Minimum voltage Vmin (pu):"; LoadFlowParameters "Load Flow parameters"
      mask help:
      | Implements a single-phase dynamic load. Active  power P and reactive
      | power Q absorbed by the load vary as function of voltage V  according to the
      | following equations:
      |
      |   If V>Vmin, P and Q vary as follows:
      |        P = Po * (V/Vo)^np * (1+Tp1.s)/(1+Tp2.s)
      |        Q = Qo * (V/Vo)^nq * (1+Tq1.s)/(1+Tq2.s)
      |   if V<Vmin
      |      Same equations with np=nq=2 (constant impedance load)
      mask init: same as IEEE34_SPSload/SM_IEEE34/DL836-1/Load B
      mask Help: helpview(psbhelp)
      mask Callback ExternalControl: powericon('ThreePhaseDynamicLoadCback',gcb);
      mask Display:
      | plot(-45,-45,45,45,[0,9,18,24,29,30,29,24,18,9,0,-9,-18,-24,-29,-30,-29,-24,-18,-9,0]*.9,[30,29,24,18,9,0,-9,-18,-24,-29,-30,-29,-24,-18,-9,0,9,18,24,29,30]*.9)
      | plot([0,0,10,0,-10,0]*1.1,[15,-5,-5,-15,-5,-5]*1.1)
  Terminator : Terminator
  In : PMIOPort  Side=Right
  wires:
  Load B/1(m) -> Terminator/1
  connections:
  In/RConn1 -- Load B/LConn1
  Load B/LConn2 -- Ground3/LConn1
